simulink model "part1"  (R2025a)
settings: Solver=ode4  StartTime=0.0  StopTime=25  FixedStep=0.1  RelTol=1e-3
values from neighbouring files (symbols this model uses):
  A = cases(c).A    [run_S1.m]    (also in run_S12_part2.m = A_list(Ai); assignin('base','A',A))
  amp = cases(c).amp    [run_S1.m]    (also in run_S12_part2.m = 1)
  b = cases(c).b    [run_S1.m]
  freq = cases(c).freq    [run_S1.m]    (also in run_S12_part2.m = 5)
  J = cases(c).J    [run_S1.m]
  theta0 = cases(c).theta0    [run_S1.m]
  useStep = cases(c).useStep    [run_S1.m]    (also in run_S12_part2.m = 1)
  w0 = cases(c).w0    [run_S1.m]
settings Model: Creator=RAJOS  LastModifiedBy=RAJOS
settings DataIOCC: SaveFormat=Array

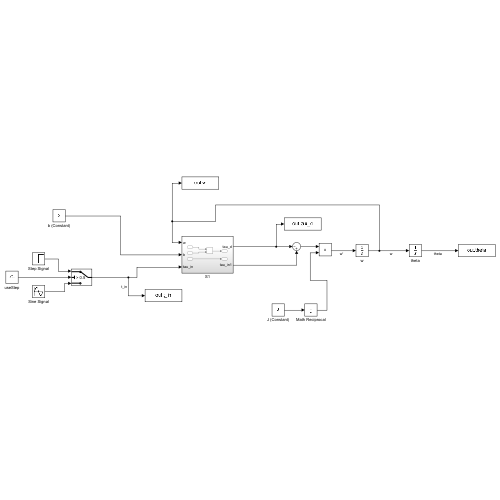
[thumbnail: Simulink's stored preview of the top-level diagram]
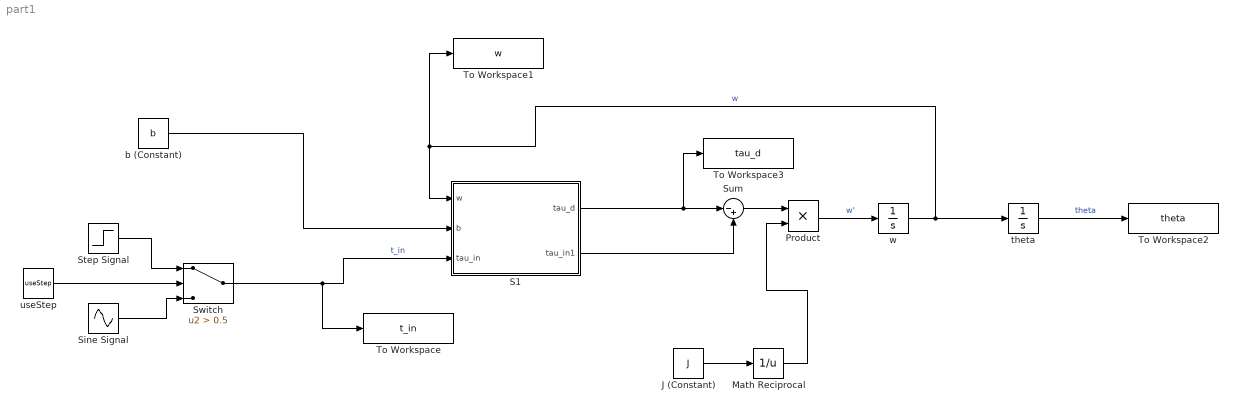
== system part1 ==
  J (Constant) : Constant  Value=J
  Math Reciprocal : Math  Operator=reciprocal  SignedPower=on
  Product : Product
  S1 : Subsystem
  Sine Signal : Sin  Amplitude=amp  Frequency=freq  SampleTime=0
  Step Signal : Step  Time=0  After=A  SampleTime=0
  Sum : Sum  Inputs=|-+
  Switch : Switch  Criteria=u2 > Threshold  Threshold=0.5  SaturateOnIntegerOverflow=off  InputSameDT=off
  To Workspace : ToWorkspace  VariableName=t_in  SampleTime=-1
  To Workspace1 : ToWorkspace  VariableName=w  SampleTime=-1
  To Workspace2 : ToWorkspace  VariableName=theta  SampleTime=-1
  To Workspace3 : ToWorkspace  VariableName=tau_d  SampleTime=-1
  b (Constant) : Constant  Value=b
  theta : Integrator  InitialCondition=theta0
  useStep : Constant  Value=useStep
  w : Integrator  InitialCondition=w0
  wires:
  w/1 -> To Workspace1/1, S1/1(w), theta/1  "w"
  theta/1 -> To Workspace2/1  "theta"
  Sine Signal/1 -> Switch/3
  Step Signal/1 -> Switch/1
  Switch/1 -> To Workspace/1, S1/3(tau_in)  "t_in"
  useStep/1 -> Switch/2
  S1/1(tau_d) -> To Workspace3/1, Sum/1
  S1/2(tau_in1) -> Sum/2
  Sum/1 -> Product/1
  Product/1 -> w/1  "w'"
  b (Constant)/1 -> S1/2(b)
  J (Constant)/1 -> Math Reciprocal/1
  Math Reciprocal/1 -> Product/2

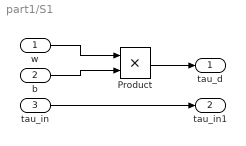
== system part1/S1 ==
  w : Inport
  b : Inport  Port=2
  tau_in : Inport  Port=3
  Product : Product
  tau_d : Outport
  tau_in1 : Outport  Port=2
  wires:
  w/1 -> Product/1
  b/1 -> Product/2
  Product/1 -> tau_d/1
  tau_in/1 -> tau_in1/1
